simulink model "SimulinkSendReceive_multiple"  (R2018a)
settings: Solver=VariableStepAuto  StartTime=0.0  StopTime=inf  RelTol=1e-3
undefined symbols (not defined in the file): LF, serial
libraries: instrumentlib x3, svdutilitieslib x1
settings Model: EnablePacing=on  Creator=Avell  LastModifiedBy=Avell

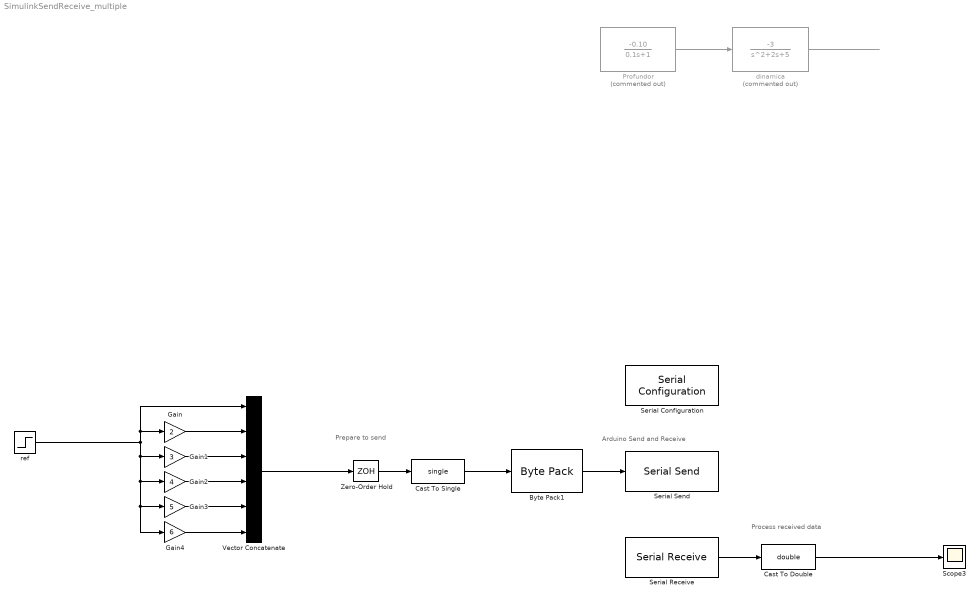
== system SimulinkSendReceive_multiple ==
  note: Process received data
  note: Prepare to send
  note: Arduino Send and Receive
  Byte Pack1 : svdutilitieslib/Byte Pack  maskPackedDataType=uint32  datatypes={'single'}  byteAlign=4  blockPlatform=arduinoert
      settings: SourceProductName=Simulink Support Package for Arduino Hardware  SourceProductBaseCode=ARDUINO
  Cast To Double : DataTypeConversion  OutDataTypeStr=double
  Cast To Single : DataTypeConversion  OutDataTypeStr=single
  Gain : Gain  Gain=2
  Gain1 : Gain  Gain=3
  Gain2 : Gain  Gain=4
  Gain3 : Gain  Gain=5
  Gain4 : Gain  Gain=6
  Profundor : TransferFcn  Commented=on  Numerator=[-0.10]  Denominator=[0.1 1]
  Scope3 : Scope
  Serial Configuration : instrumentlib/Serial Configuration  Priority=-200000  ComPortMenu=<Please select a port...>  ComPort=COM15  ObjConstructor=serial('COM15');  BaudRate=115200  DataBits=8  Parity=none  StopBits=1  FlowControl=none  Timeout=10  ByteOrder=LittleEndian
  Serial Receive : instrumentlib/Serial Receive  ComPortMenu=<Please select a port...>  ComPort=COM15  ObjConstructor=serial('COM15');  Header=A  Terminator=LF ('\n')  DataSize="[1  3]"  DataType=single  EnableBlockingMode=on  ActionDataUnavailable=Output last received value  CustomValue=0  SampleTime=0.05
  Serial Send : instrumentlib/Serial Send  ComPortMenu=<Please select a port...>  ComPort=COM15  ObjConstructor=serial('COM15');  Terminator=<none>  EnableBlockingMode=on
  Vector Concatenate : Concatenate  NumInputs=6
  Zero-Order Hold : ZeroOrderHold  SampleTime=0.05
  dinamica : TransferFcn  Commented=on  Numerator=[-3]  Denominator=[1 2 5]
  ref : Step  SampleTime=0.1
  wires:
  Profundor/1 -> dinamica/1
  ref/1 -> Gain/1, Vector Concatenate/1, Gain4/1, Gain3/1, Gain2/1, Gain1/1
  dinamica/1 -> ?
  Vector Concatenate/1 -> Zero-Order Hold/1
  Gain/1 -> Vector Concatenate/2
  Gain1/1 -> Vector Concatenate/3
  Gain2/1 -> Vector Concatenate/4
  Gain3/1 -> Vector Concatenate/5
  Gain4/1 -> Vector Concatenate/6
  Cast To Single/1 -> Byte Pack1/1
  Byte Pack1/1 -> Serial Send/1
  Serial Receive/1 -> Cast To Double/1
  Zero-Order Hold/1 -> Cast To Single/1
  Cast To Double/1 -> Scope3/1
